simulink model "AccurateSimulation"  (R2020b)
settings: Solver=ode45  StartTime=0.0  StopTime=35  RelTol=1e-3
values from neighbouring files (symbols this model uses):
  deg2pulse = 1/pulse2deg    (= 11.3777777778)    [LoadParameters.m]
  Kd = Kp * Td    [DesignPIDBode.m]    (also in DesignPIDProgrammatically.m = 0)
  Kdrv = ((R3+R4)*R2)/(R4*(R1+R2))    (= 0.597802197802)    [LoadParameters.m]
  Ke = 7.68e-3    (= 0.00768)    [LoadParameters.m]
  Keq = 1/Beq    (= 500000)    [LoadParameters.m]
  Ki = Kp / Ti    [DesignPIDBode.m]    (also in DesignPIDProgrammatically.m = 0)
  Kmot = 1/(Rs+Ra)    (= 0.322580645161)    [LoadParameters.m]
  Kp = DeltaK * cosd(DeltaPhi)    [DesignPIDBode.m]    (also in DesignPIDProgrammatically.m = 0)
  Kt = 7.68e-3    (= 0.00768)    [EstimateBeq_tausf.m]    (also in EstimateJeq.m; LS.m; LoadParameters.m)
  N = 14    [EstimateBeq_tausf.m]    (also in EstimateJeq.m; LS.m; LoadParameters.m)
  pulse2deg = enc_step    (= 0.087890625)    [LoadParameters.m]
  rad2rpm = 60/2/pi    (= 9.54929658551)    [LoadParameters.m]
  tausf = b*Kt*Rs*N    [EstimateBeq_tausf.m]    (also in EstimateJeq.m = 0.00909; LS.m; LoadParameters.m = 0.01)
  Tdrv = (R1*R2*C1)/(R1+R2)    (= 0.000131868131868)    [LoadParameters.m]
  Teq = Jeq/Beq    (= 0.282244897959)    [LoadParameters.m]
  Tmot = La/(Rs+Ra)    (= 5.8064516129e-05)    [LoadParameters.m]
  Tsample = 1e-3    (= 0.001)    [EstimateBeq_tausf.m]    (also in EstimateJeq.m; LS.m; LoadParameters.m)
  vcc = -10    [LoadParameters.m]
  vdd = 10    [LoadParameters.m]
  vm = -12    [LoadParameters.m]
  vp = 12    [LoadParameters.m]
libraries: simulink x1
settings Model: Creator=Utente  LastModifiedBy=Utente
settings SolverCC: ZeroCrossAlgorithm=Adaptive
settings DebuggingCC: IgnoredZcDiagnostic=none

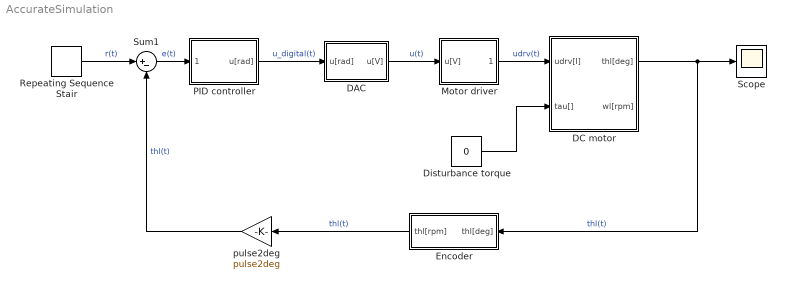
== system AccurateSimulation ==
  DAC : Subsystem
  DC motor : Subsystem
  Disturbance torque : Constant  Value=0
  Encoder : Subsystem
  Motor driver : Subsystem
  PID controller : Subsystem
  Repeating Sequence Stair : simulink/Sources/Repeating Sequence Stair  OutValues=[0 10 30 50 90 180 360]  tsamp=5  OutMin=[]  OutMax=[]  OutDataTypeStr=double  OutputDataTypeScalingMode=double  OutDataType=fixdt(0,8)  ConRadixGroup=Best Precision: Vector-wise  OutScaling=2^-12
  Scope : Scope
  Sum1 : Sum  Inputs=|+-
  pulse2deg : Gain  Gain=pulse2deg
  wires:
  Motor driver/1(udrv[I]) -> DC motor/1(udrv[I])  "udrv(t)"
  DAC/1(u[V]) -> Motor driver/1(u[V])  "u(t)"
  Encoder/1(thl[rpm]) -> pulse2deg/1  "thl(t)"
  pulse2deg/1 -> Sum1/2  "thl(t)"
  Sum1/1 -> PID controller/1(e[deg])  "e(t)"
  PID controller/1(u[rad]) -> DAC/1(u[rad])  "u_digital(t)"
  DC motor/1(thl[deg]) -> Scope/1, Encoder/1(thl[deg])  "thl(t)"
  Repeating Sequence Stair/1 -> Sum1/1  "r(t)"
  Disturbance torque/1 -> DC motor/2(tau[])

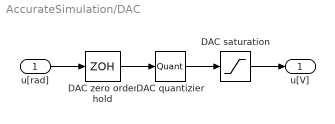
== system AccurateSimulation/DAC ==
  u[rad] : Inport
  DAC quantizier : Quantizer  QuantizationInterval=q_step
  DAC saturation : Saturate  UpperLimit=vdd  LowerLimit=vcc
  DAC zero order hold : ZeroOrderHold  SampleTime=Tsample
  u[V] : Outport
  wires:
  DAC quantizier/1 -> DAC saturation/1
  DAC zero order hold/1 -> DAC quantizier/1
  DAC saturation/1 -> u[V]/1
  u[rad]/1 -> DAC zero order hold/1

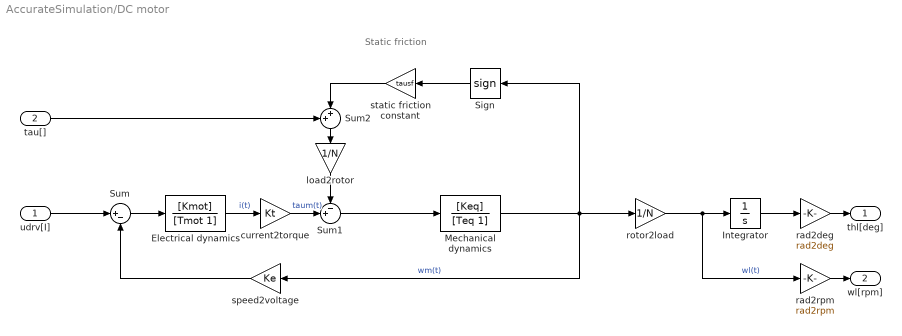
== system AccurateSimulation/DC motor ==
  note: Static friction
  udrv[I] : Inport  Unit=V
  tau[] : Inport  Port=2  Unit=V
  Electrical dynamics : TransferFcn  Numerator=[Kmot]  Denominator=[Tmot 1]
  Integrator : Integrator
  Mechanical dynamics : TransferFcn  Numerator=[Keq]  Denominator=[Teq 1]
  Sign : Signum  ZeroCross=off
  Sum : Sum  Inputs=|+-
  Sum1 : Sum  Inputs=-+|
  Sum2 : Sum  Inputs=++|
  current2torque : Gain  Gain=Kt
  load2rotor : Gain  Gain=1/N
  rad2deg : Gain  Gain=rad2deg
  rad2rpm : Gain  Gain=rad2rpm
  rotor2load : Gain  Gain=1/N
  speed2voltage : Gain  Gain=Ke
  static friction constant : Gain  Gain=tausf
  thl[deg] : Outport  Unit=deg
  wl[rpm] : Outport  Port=2  Unit=rpm
  wires:
  load2rotor/1 -> Sum1/1
  Mechanical dynamics/1 -> Sign/1, rotor2load/1, speed2voltage/1  "wm(t)"
  Sign/1 -> static friction constant/1
  current2torque/1 -> Sum1/2  "taum(t)"
  Sum1/1 -> Mechanical dynamics/1
  speed2voltage/1 -> Sum/2
  rotor2load/1 -> rad2rpm/1, Integrator/1  "wl(t)"
  Electrical dynamics/1 -> current2torque/1  "i(t)"
  Integrator/1 -> rad2deg/1
  Sum/1 -> Electrical dynamics/1
  rad2rpm/1 -> wl[rpm]/1
  rad2deg/1 -> thl[deg]/1
  udrv[I]/1 -> Sum/1
  static friction constant/1 -> Sum2/2
  Sum2/1 -> load2rotor/1
  tau[]/1 -> Sum2/1

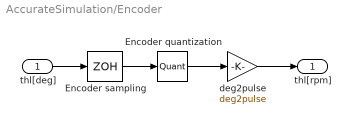
== system AccurateSimulation/Encoder ==
  thl[deg] : Inport
  Encoder quantization : Quantizer  QuantizationInterval=enc_step
  Encoder sampling : ZeroOrderHold  SampleTime=Tsample
  deg2pulse : Gain  Gain=deg2pulse
  thl[rpm] : Outport
  wires:
  Encoder quantization/1 -> deg2pulse/1
  deg2pulse/1 -> thl[rpm]/1
  Encoder sampling/1 -> Encoder quantization/1
  thl[deg]/1 -> Encoder sampling/1

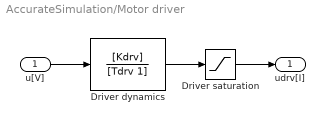
== system AccurateSimulation/Motor driver ==
  u[V] : Inport
  Driver dynamics : TransferFcn  Numerator=[Kdrv]  Denominator=[Tdrv 1]
  Driver saturation : Saturate  UpperLimit=vp  LowerLimit=vm
  udrv[I] : Outport
  wires:
  Driver saturation/1 -> udrv[I]/1
  Driver dynamics/1 -> Driver saturation/1
  u[V]/1 -> Driver dynamics/1

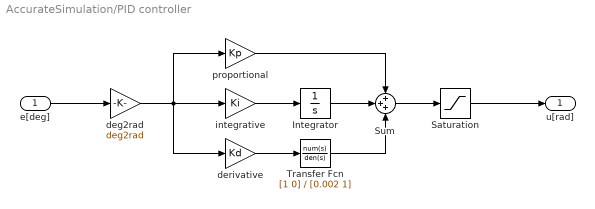
== system AccurateSimulation/PID controller ==
  e[deg] : Inport  Unit=deg
  Integrator : Integrator
  Saturation : Saturate  UpperLimit=vdd  LowerLimit=vcc
  Sum : Sum  Inputs=+++
  Transfer Fcn : TransferFcn  Numerator=[1 0]  Denominator=[0.002 1]
  deg2rad : Gain  Gain=deg2rad
  derivative : Gain  Gain=Kd
  integrative : Gain  Gain=Ki
  proportional : Gain  Gain=Kp
  u[rad] : Outport
  wires:
  e[deg]/1 -> deg2rad/1
  Sum/1 -> Saturation/1
  Transfer Fcn/1 -> Sum/3
  deg2rad/1 -> proportional/1, derivative/1, integrative/1
  proportional/1 -> Sum/1
  integrative/1 -> Integrator/1
  Integrator/1 -> Sum/2
  Saturation/1 -> u[rad]/1
  derivative/1 -> Transfer Fcn/1
